simulink model "rectifier"  (R2024b)
settings: Solver=VariableStepAuto  StartTime=0.0  StopTime=10.0  RelTol=1e-3
settings Model: Creator=rohan  LastModifiedBy=rohan

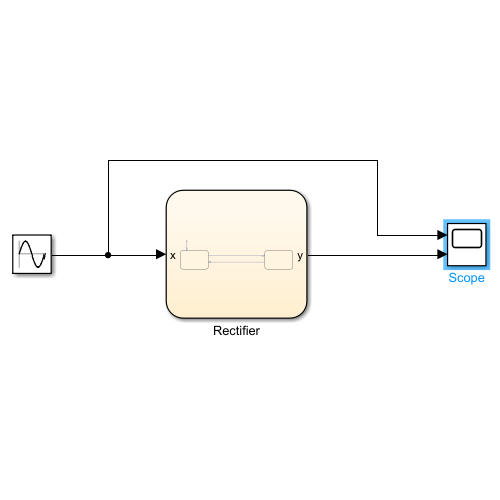
[thumbnail: Simulink's stored preview of the top-level diagram]
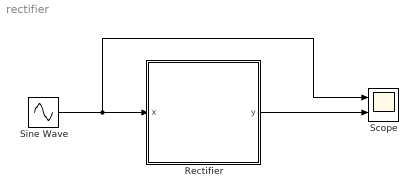
== system rectifier ==
  Rectifier : Stateflow chart  TreatAsAtomicUnit=on
  Scope : Scope  NumInputPorts=2
  Sine Wave : Sin  SampleTime=0
  wires:
  Sine Wave/1 -> Scope/1, Rectifier/1(x)
  Rectifier/1(y) -> Scope/2

== stateflow chart rectifier/Rectifier ==
  state ON
    y=x;
  state OFF
    y=0;
  (default) -> ON
  ON -> OFF : [x<t0]
  OFF -> ON : [x>=t0]
  data: x input; y output; t0 constant double
